simulink model "Final_Reciprocating_Simscape_19_08_24"  (R2023b)
settings: Solver=FixedStepAuto  StartTime=0.0  StopTime=T(end)  FixedStep=10^-4  RelTol=1e-3
values from neighbouring files (symbols this model uses):
  Kp1 = 10    [FFFB_PosForce_ME.m]    (also in FFFB_PosForce_ME1.m = 5000; FFFB_PosForce_ME2.m = 5000; FFFB_Posarbitary_actual_Mass.m = 5000; FFFB_arbitary_actual_Mass.m = 5000)
  Kp2 = 10000    [FFFB_PosForce_ME1.m]    (also in FFFB_PosForce_ME2.m; FFFB_Posarbitary_actual_Mass.m; FFFB_arbitary_actual_Mass.m; Kin_Trajectory_23_09_24.m)
  N = [-y1+y3;-x3+x1]    [Contact.m]
  X = 0.65    [Contact.m]    (also in FFFB_PosForce_ME.m = [X0',X1',X2']; FFFB_PosForce_ME1.m = [X2']; FFFB_PosForce_ME2.m = [X110,X2']; FFFB_Posarbitary_actual_Mass.m = [X110])
  Y = [Y0',Y1',Y2']    [FFFB_PosForce_ME.m]    (also in FFFB_PosForce_ME1.m = [Y2']; FFFB_PosForce_ME2.m = [Y110,Y2']; FFFB_Posarbitary_actual_Mass.m = [Y110]; FFFB_arbitary_actual_Mass.m = [Y2'])
undefined symbols (not defined in the file or in its folder): Z
libraries: sm_lib x24, nesl_utility x9, robotcorelib x1
settings Model: Creator=91996  LastModifiedBy=Dell
settings ExplorerConfigSet: InternalSimMechanicsExplorerSettings="<ExplorerConfiguration><canonicalview>default</canonicalview><AnimationSetting><BasePlaybackSpeed>1.0</BasePlaybackSpeed><PlaybackSpeedFactor>256.0</PlaybackSpeedFactor></AnimationSetting><TilePanel><TileInfo><Tiles Columns=\"1\" Count=\"1\" Rows=\"1\"><Column Weight=\"1\"/><Row Weight=\"1\"/><Tile Height=\"1\" Width=\"1\" X=\"0\" Y=\"0\"/></Tiles></TileInfo><SceneInfo><SceneViewer><BGColor><R>0.941176474094390869</R><G>0.941176474094390869</G><B>0.941176474094390869</B></BGColor><Camera><DoPerspective>off</DoPerspective><Position><X>0.490000009536743164</X><Y>-0.75</Y><Z>0.0764452517032630507</Z></Position><Center><X>0.490000009536743164</X><Y>0.25</Y><Z>0.0764452517032630507</Z></Center><Up><X>0</X><Y>-0</Y><Z>1</Z></Up><ViewLimDist>1</ViewLimDist><YLim>0.35683862030506136</YLim><XLim>0.73638515281135386</XLim></Camera></SceneViewer></SceneInfo></TilePanel><MechEditorPanel><Cameras/><GfxPanelCameraMap/><VideoCreator><PlaybackSpeedRatio>1.0</PlaybackSpeedRatio><FrameRate>30</FrameRate><VideoFormat>Motion JPEG AVI</VideoFormat><FrameSize>auto</FrameSize></VideoCreator></MechEditorPanel></ExplorerConfiguration>"

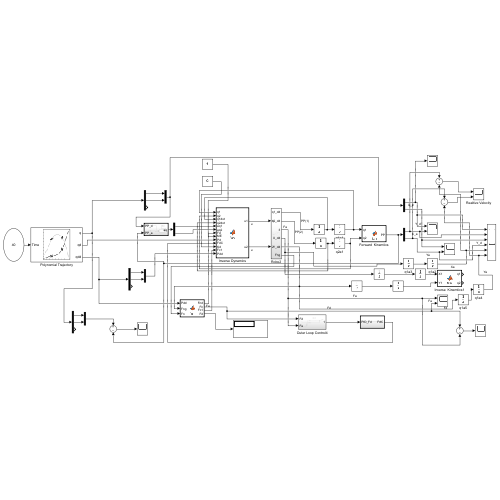
[thumbnail: Simulink's stored preview of the top-level diagram]
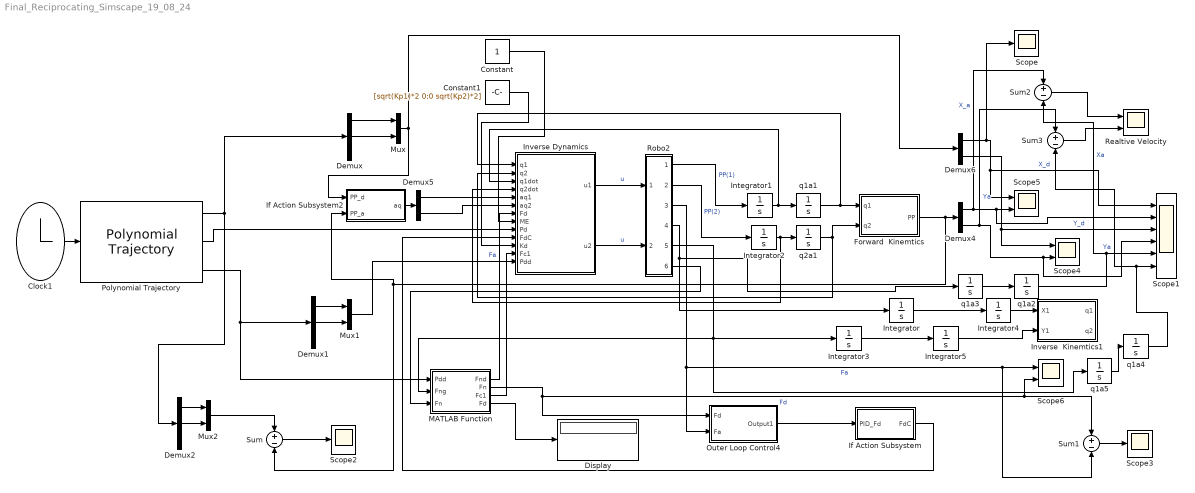
== system Final_Reciprocating_Simscape_19_08_24 ==
  Clock1 : Clock
  Constant : Constant
  Constant1 : Constant  Value=[sqrt(Kp1)*2 0;0 sqrt(Kp2)*2]
  Demux : Demux  Outputs=3
  Demux1 : Demux  Outputs=3
  Demux2 : Demux  Outputs=3
  Demux4 : Demux  Outputs=2
  Demux5 : Demux  Outputs=2
  Demux6 : Demux  Outputs=2
  Display : Display
  Forward  Kinemtics : MATLAB Function  TreatAsAtomicUnit=on
  If Action Subsystem : Subsystem  TreatAsAtomicUnit=on
  If Action Subsystem2 : Subsystem  TreatAsAtomicUnit=on
  Integrator{,1..5} (6 alike) : Integrator
  Inverse  Kinemtics1 : MATLAB Function  TreatAsAtomicUnit=on
  Inverse Dynamics : MATLAB Function  TreatAsAtomicUnit=on
  MATLAB Function : MATLAB Function  TreatAsAtomicUnit=on
  Mux : Mux  Inputs=2
  Mux1 : Mux  Inputs=2
  Mux2 : Mux  Inputs=2
  Outer Loop Control4 : Subsystem
  Polynomial Trajectory : robotcorelib/Polynomial Trajectory  WaypointSource=Internal  Waypoints=P  TimePoints=T  TimeInterval=[ 1, 4 ]  Method=Quintic Polynomial  ParameterSource=Internal  VelocityBoundaryCondition=Pd  AccelerationBoundaryCondition=Pdd  SimulateUsing=Interpreted execution
  Realtive Velocity : Scope  NumInputPorts=2
  Robo2 : Subsystem
  Scope : Scope
  Scope1 : Scope  NumInputPorts=6
  Scope2 : Scope
  Scope3 : Scope
  Scope4 : Scope  NumInputPorts=2
  Scope5 : Scope  NumInputPorts=2
  Scope6 : Scope  NumInputPorts=2
  Sum{,1..3} (4 alike) : Sum  Inputs=+-
  q1a1 : Integrator  InitialCondition=0.3778
  q1a2 : Integrator  InitialCondition=0.65
  q1a3 : Integrator
  q1a4 : Integrator  InitialCondition=0.2
  q1a5 : Integrator
  q2a1 : Integrator  InitialCondition=-1.5690
  wires:
  Inverse Dynamics/1(u1) -> Robo2/1(Input)  "u"
  Demux5/2 -> Inverse Dynamics/6(aq2)
  Demux6/2 -> Scope4/1, Scope1/3  "Y_d"
  Mux/1 -> If Action Subsystem2/1(PP_d), Demux6/1
  Integrator4/1 -> Inverse  Kinemtics1/1(X1)
  Robo2/5(Y_dd) -> q1a5/1, Integrator3/1, MATLAB Function/2(Fng)
  Demux/1 -> Mux/1
  Integrator/1 -> Integrator4/1
  Integrator3/1 -> Integrator5/1
  Integrator5/1 -> Inverse  Kinemtics1/2(Y1)
  Demux5/1 -> Inverse Dynamics/5(aq1)
  Polynomial Trajectory/3 -> MATLAB Function/1(Pdd), Demux1/1
  Demux4/1 -> Sum2/1, Scope1/2, Scope5/2  "X_a"
  If Action Subsystem2/1(aq) -> Demux5/1
  Clock1/1 -> Polynomial Trajectory/1
  q2a1/1 -> Forward  Kinemtics/2(q2), Inverse Dynamics/2(q2)
  Outer Loop Control4/1(Output1) -> If Action Subsystem/1(PID_Fd)
  Robo2/4(X_dd) -> q1a3/1, Integrator/1
  Integrator2/1 -> q2a1/1, Inverse Dynamics/4(q2dot)
  Demux6/1 -> Scope/1, Scope5/1, Scope1/1  "X_d"
  Inverse Dynamics/2(u2) -> Robo2/2(Input1)  "u"
  Integrator1/1 -> q1a1/1, Inverse Dynamics/3(q1dot)
  Robo2/2(q2_dd) -> Integrator2/1  "PP(2)"
  q1a1/1 -> Forward  Kinemtics/1(q1), Inverse Dynamics/1(q1)
  Robo2/1(q1_dd) -> Integrator1/1  "PP(1)"
  Demux/2 -> Mux/2
  Demux4/2 -> Scope1/4, Scope4/2, Sum3/1  "Ya"
  Constant/1 -> Inverse Dynamics/8(ME)
  Mux2/1 -> Sum/1
  Forward  Kinemtics/1(PP) -> Sum/2, If Action Subsystem2/2(PP_a), Demux4/1
  Sum/1 -> Scope2/1
  Demux2/2 -> Mux2/2
  Polynomial Trajectory/1 -> Demux/1, Demux2/1
  Demux2/1 -> Mux2/1
  MATLAB Function/2(Fn) -> Outer Loop Control4/1(Fd), Scope6/2, Sum1/1  "Fd"
  Sum1/1 -> Scope3/1
  Robo2/3(Output2) -> Outer Loop Control4/2(Fa), Scope6/1, Sum1/2  "Fa"
  Polynomial Trajectory/2 -> Inverse Dynamics/9(Pd)
  If Action Subsystem/1(FdC) -> Inverse Dynamics/10(FdC)
  Constant1/1 -> Inverse Dynamics/11(Kd)
  MATLAB Function/1(Fnd) -> Inverse Dynamics/7(Fd)  "Fa"
  MATLAB Function/3(Fc1) -> Inverse Dynamics/12(Fc1)
  Demux1/1 -> Mux1/1
  Demux1/2 -> Mux1/2
  Mux1/1 -> Inverse Dynamics/13(Pdd)
  Robo2/6(Fng) -> MATLAB Function/3("Fn ")
  MATLAB Function/4(Fd) -> Display/1
  q1a3/1 -> q1a2/1
  q1a2/1 -> Sum2/2, Scope1/5  "Xa"
  q1a5/1 -> q1a4/1
  q1a4/1 -> Sum3/2, Scope1/6  "Ya"
  Sum2/1 -> Realtive Velocity/1
  Sum3/1 -> Realtive Velocity/2

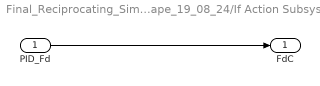
== system Final_Reciprocating_Simscape_19_08_24/If Action Subsystem ==
  PID_Fd : Inport
  FdC : Outport
  wires:
  PID_Fd/1 -> FdC/1

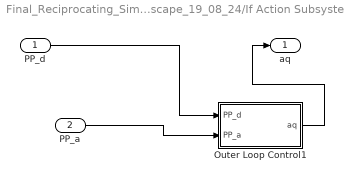
== system Final_Reciprocating_Simscape_19_08_24/If Action Subsystem2 ==
  PP_d : Inport
  PP_a : Inport  Port=2
  Outer Loop Control1 : Subsystem
  aq : Outport
  wires:
  PP_d/1 -> Outer Loop Control1/1(PP_d)
  Outer Loop Control1/1(aq) -> aq/1
  PP_a/1 -> Outer Loop Control1/2(PP_a)

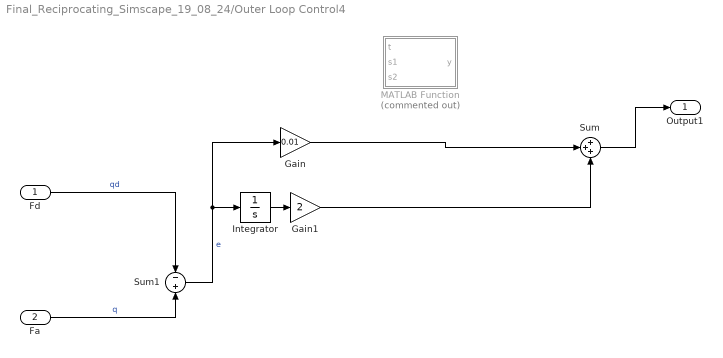
== system Final_Reciprocating_Simscape_19_08_24/Outer Loop Control4 ==
  Fd : Inport
  Fa : Inport  Port=2
  Gain : Gain  Gain=0.01
  Gain1 : Gain  Gain=2
  Integrator : Integrator
  MATLAB Function : MATLAB Function  Commented=on  TreatAsAtomicUnit=on
  Sum : Sum  Inputs=+++
  Sum1 : Sum  Inputs=-+
  Output1 : Outport
  wires:
  Sum1/1 -> Gain/1, Integrator/1  "e"
  Fd/1 -> Sum1/1  "qd"
  Fa/1 -> Sum1/2  "q"
  Integrator/1 -> Gain1/1
  Gain/1 -> Sum/2
  Gain1/1 -> Sum/3
  Sum/1 -> Output1/1

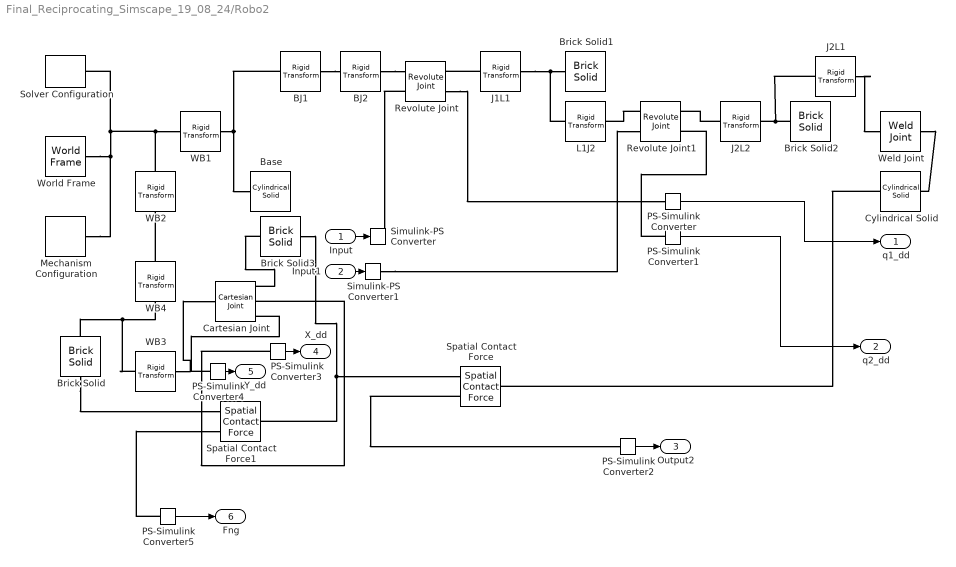
== system Final_Reciprocating_Simscape_19_08_24/Robo2 ==
  Input : Inport
  Input1 : Inport  Port=2
  BJ1 : sm_lib/Frames and Transforms/Rigid Transform  TranslationMethod=StandardAxis  TranslationStandardOffset=0.25  TranslationStandardOffsetUnits=m  TranslationStandardAxis=+Z  TranslationCartesianOffset=[0 0 0]  TranslationCartesianOffsetUnits=m  TranslationROffset=0  TranslationROffsetUnits=m  TranslationZOffset=0  TranslationZOffsetUnits=m  TranslationThetaOffset=0  TranslationThetaOffsetUnits=deg  RotationMethod=StandardAxis  RotationAngleUnits=deg  RotationStandardAxis=+X  RotationAngle=90  RotationArbitraryAxis=[0 0 1]  FollAlignAxisA=+X  BaseAlignAxisA=+Y  FollAlignAxisB=+Y  BaseAlignAxisB=+Z  RotationSequenceAxes=FollowerAxes  RotationSequence=XYX  RotationSequenceAngles=[0 0 0]  RotationSequenceAnglesUnits=deg  RotationMatrix=[1 0 0; 0 1 0; 0 0 1]  Quaternion=[1 0 0 0]
  BJ2 : sm_lib/Frames and Transforms/Rigid Transform  TranslationMethod=None  TranslationStandardOffset=0  TranslationStandardOffsetUnits=m  TranslationStandardAxis=+Z  TranslationCartesianOffset=[0 0 0]  TranslationCartesianOffsetUnits=m  TranslationROffset=0  TranslationROffsetUnits=m  TranslationZOffset=0  TranslationZOffsetUnits=m  TranslationThetaOffset=0  TranslationThetaOffsetUnits=deg  RotationMethod=StandardAxis  RotationAngleUnits=rad  RotationStandardAxis=+Z  RotationAngle=0.3778  RotationArbitraryAxis=[0 0 1]  FollAlignAxisA=+X  BaseAlignAxisA=+Y  FollAlignAxisB=+Y  BaseAlignAxisB=+Z  RotationSequenceAxes=FollowerAxes  RotationSequence=XYX  RotationSequenceAngles=[0 0 0]  RotationSequenceAnglesUnits=deg  RotationMatrix=[1 0 0; 0 1 0; 0 0 1]  Quaternion=[1 0 0 0]
  Base : sm_lib/Body Elements/Cylindrical Solid  GraphicAmbientColor=[0.15 0.15 0.15 1.0]  BasedOnType=Density  CenterOfMass=[0 0 0]  CenterOfMassUnits=m  GraphicDiffuseColor=[0.5 0.5 0.5]  CylinderLength=0.5  CylinderLengthUnits=m  CylinderRadius=0.02  CylinderRadiusUnits=m  Density=10000  DensityUnits=kg/m^3  DoExposeReferenceFrame=on  GraphicEmissiveColor=[0.0 0.0 0.0 1.0]  ExportEntireGeometry=off  SerializedFrames=<Frames/>  MarkerShape=Sphere  MarkerSize=10  GraphicType=FromGeometry  InertiaType=CalculateFromGeometry  Mass=1  MassUnits=kg  MomentsOfInertia=[1 1 1]  MomentsOfInertiaUnits=kg*m^2  GraphicOpacity=1.0  ProductsOfInertia=[0 0 0]  ProductsOfInertiaUnits=kg*m^2  GraphicShininess=75  GraphicSpecularColor=[0.5 0.5 0.5 1.0]  GraphicVisPropType=SimpleVisualProperties
  Brick Solid : sm_lib/Body Elements/Brick Solid  GraphicAmbientColor=[0.15 0.15 0.15 1.0]  BasedOnType=Density  BrickDimensions=[1 0.02 0.02]  BrickDimensionsUnits=m  CenterOfMass=[0 0 0]  CenterOfMassUnits=m  GraphicDiffuseColor=[0.5 0.5 0.5]  Density=10000  DensityUnits=kg/m^3  DoExposeReferenceFrame=on  GraphicEmissiveColor=[0.0 0.0 0.0 1.0]  ExportEntireGeometry=on  SerializedFrames=<Frames/>  MarkerShape=Sphere  MarkerSize=10  GraphicType=FromGeometry  InertiaType=CalculateFromGeometry  Mass=1  MassUnits=kg  MomentsOfInertia=[1 1 1]  MomentsOfInertiaUnits=kg*m^2  GraphicOpacity=1.0  ProductsOfInertia=[0 0 0]  ProductsOfInertiaUnits=kg*m^2  GraphicShininess=75  GraphicSpecularColor=[0.5 0.5 0.5 1.0]  GraphicVisPropType=SimpleVisualProperties
  Brick Solid1 : sm_lib/Body Elements/Brick Solid  GraphicAmbientColor=[0.15 0.15 0.15 1.0]  BasedOnType=Density  BrickDimensions=[0.5 0.02 0.02]  BrickDimensionsUnits=m  CenterOfMass=[0 0 0]  CenterOfMassUnits=m  GraphicDiffuseColor=[0.2 0.2 1.0]  Density=7800  DensityUnits=kg/m^3  DoExposeReferenceFrame=on  GraphicEmissiveColor=[0.0 0.0 0.0 1.0]  ExportEntireGeometry=off  SerializedFrames=<Frames/>  MarkerShape=Sphere  MarkerSize=10  GraphicType=FromGeometry  InertiaType=CalculateFromGeometry  Mass=1  MassUnits=kg  MomentsOfInertia=[1 1 1]  MomentsOfInertiaUnits=kg*m^2  GraphicOpacity=1.0  ProductsOfInertia=[0 0 0]  ProductsOfInertiaUnits=kg*m^2  GraphicShininess=75  GraphicSpecularColor=[0.5 0.5 0.5 1.0]  GraphicVisPropType=SimpleVisualProperties
  Brick Solid2 : sm_lib/Body Elements/Brick Solid  GraphicAmbientColor=[0.15 0.15 0.15 1.0]  BasedOnType=Density  BrickDimensions=[0.5 0.02 0.02]  BrickDimensionsUnits=m  CenterOfMass=[0 0 0]  CenterOfMassUnits=m  GraphicDiffuseColor=[0.0 0.8 0.2]  Density=7800  DensityUnits=kg/m^3  DoExposeReferenceFrame=on  GraphicEmissiveColor=[0.0 0.0 0.0 1.0]  ExportEntireGeometry=off  SerializedFrames=<Frames/>  MarkerShape=Sphere  MarkerSize=10  GraphicType=FromGeometry  InertiaType=CalculateFromGeometry  Mass=1  MassUnits=kg  MomentsOfInertia=[1 1 1]  MomentsOfInertiaUnits=kg*m^2  GraphicOpacity=1.0  ProductsOfInertia=[0 0 0]  ProductsOfInertiaUnits=kg*m^2  GraphicShininess=75  GraphicSpecularColor=[0.5 0.5 0.5 1.0]  GraphicVisPropType=SimpleVisualProperties
  Brick Solid3 : sm_lib/Body Elements/Brick Solid  GraphicAmbientColor=[0.15 0.15 0.15 1.0]  BasedOnType=Density  BrickDimensions=[0.22 0.02 0.2]  BrickDimensionsUnits=m  CenterOfMass=[0 0 0]  CenterOfMassUnits=m  GraphicDiffuseColor=[1.0 0.2 0.2]  Density=2000  DensityUnits=kg/m^3  DoExposeReferenceFrame=on  GraphicEmissiveColor=[0.0 0.0 0.0 1.0]  ExportEntireGeometry=on  SerializedFrames=<Frames/>  MarkerShape=Sphere  MarkerSize=10  GraphicType=FromGeometry  InertiaType=CalculateFromGeometry  Mass=1  MassUnits=kg  MomentsOfInertia=[1 1 1]  MomentsOfInertiaUnits=kg*m^2  GraphicOpacity=1.0  ProductsOfInertia=[0 0 0]  ProductsOfInertiaUnits=kg*m^2  GraphicShininess=75  GraphicSpecularColor=[0.5 0.5 0.5 1.0]  GraphicVisPropType=SimpleVisualProperties
  Cartesian Joint : sm_lib/Joints/Cartesian Joint  JointMode=Normal  SenseConstraintForce=off  SenseConstraintForceX=off  SenseConstraintForceY=off  SenseConstraintForceZ=off  SenseConstraintTorque=off  SenseConstraintTorqueX=off  SenseConstraintTorqueY=off  SenseConstraintTorqueZ=off  SenseTotalForce=off  SenseTotalForceX=off  SenseTotalForceY=off  SenseTotalForceZ=off  SenseTotalTorque=off  SenseTotalTorqueX=off  SenseTotalTorqueY=off  SenseTotalTorqueZ=off  CompositeWrenchDir=FollowerOnBase  CompositeWrenchFrame=BaseFrame  PxEquilibriumPosition=0  PxEquilibriumPositionUnits=m  PxSpringStiffness=0  PxSpringStiffnessUnits=N/m  PxDampingCoefficient=0  PxDampingCoefficientUnits=N/(m/s)  PxTorqueActuationMode=NoTorque  PxMotionActuationMode=ComputedMotion  PxSensePosition=off  PxSenseVelocity=off  PxSenseAcceleration=on  PxSenseTorqueForce=off  PxSenseLowerLimitTorqueForce=off  PxSenseUpperLimitTorqueForce=off  PxLowerLimitSpecify=off  PxLowerLimitBound=-1  PxLowerLimitBoundUnits=m  PxLowerLimitStiffness=1e6  PxLowerLimitStiffnessUnits=N/m  PxLowerLimitDamping=1e3  PxLowerLimitDampingUnits=N/(m/s)  PxLowerLimitTransitionRegionWidth=1e-4  PxLowerLimitTransitionRegionWidthUnits=m  PxUpperLimitSpecify=off  PxUpperLimitBound=1  PxUpperLimitBoundUnits=m  PxUpperLimitStiffness=1e6  PxUpperLimitStiffnessUnits=N/m  PxUpperLimitDamping=1e3  PxUpperLimitDampingUnits=N/(m/s)  PxUpperLimitTransitionRegionWidth=1e-4  PxUpperLimitTransitionRegionWidthUnits=m  PxPositionTargetSpecify=off  PxPositionTargetPriority=High  PxPositionTargetValue=0  PxPositionTargetValueUnits=m  PxVelocityTargetSpecify=off  PxVelocityTargetPriority=High  PxVelocityTargetValue=0  PxVelocityTargetValueUnits=m/s  PyEquilibriumPosition=0  PyEquilibriumPositionUnits=m  PySpringStiffness=0  PySpringStiffnessUnits=N/m  PyDampingCoefficient=0  PyDampingCoefficientUnits=N/(m/s)  PyTorqueActuationMode=NoTorque  PyMotionActuationMode=ComputedMotion  PySensePosition=off  PySenseVelocity=off  PySenseAcceleration=off  PySenseTorqueForce=off  PySenseLowerLimitTorqueForce=off  PySenseUpperLimitTorqueForce=off  PyLowerLimitSpecify=off  PyLowerLimitBound=-1  PyLowerLimitBoundUnits=m  PyLowerLimitStiffness=1e6  PyLowerLimitStiffnessUnits=N/m  PyLowerLimitDamping=1e3  PyLowerLimitDampingUnits=N/(m/s)  PyLowerLimitTransitionRegionWidth=1e-4  PyLowerLimitTransitionRegionWidthUnits=m  PyUpperLimitSpecify=off  PyUpperLimitBound=1  PyUpperLimitBoundUnits=m  PyUpperLimitStiffness=1e6  PyUpperLimitStiffnessUnits=N/m  PyUpperLimitDamping=1e3  PyUpperLimitDampingUnits=N/(m/s)  PyUpperLimitTransitionRegionWidth=1e-4  PyUpperLimitTransitionRegionWidthUnits=m  PyPositionTargetSpecify=off  PyPositionTargetPriority=High  PyPositionTargetValue=0  PyPositionTargetValueUnits=m  PyVelocityTargetSpecify=off  PyVelocityTargetPriority=High  PyVelocityTargetValue=0  PyVelocityTargetValueUnits=m/s  PzEquilibriumPosition=0  PzEquilibriumPositionUnits=m  PzSpringStiffness=0  PzSpringStiffnessUnits=N/m  PzDampingCoefficient=0  PzDampingCoefficientUnits=N/(m/s)  PzTorqueActuationMode=NoTorque  PzMotionActuationMode=ComputedMotion  PzSensePosition=off  PzSenseVelocity=off  PzSenseAcceleration=on  PzSenseTorqueForce=off  PzSenseLowerLimitTorqueForce=off  PzSenseUpperLimitTorqueForce=off  PzLowerLimitSpecify=off  PzLowerLimitBound=-1  PzLowerLimitBoundUnits=m  PzLowerLimitStiffness=1e6  PzLowerLimitStiffnessUnits=N/m  PzLowerLimitDamping=1e3  PzLowerLimitDampingUnits=N/(m/s)  PzLowerLimitTransitionRegionWidth=1e-4  PzLowerLimitTransitionRegionWidthUnits=m  PzUpperLimitSpecify=off  PzUpperLimitBound=1  PzUpperLimitBoundUnits=m  PzUpperLimitStiffness=1e6  PzUpperLimitStiffnessUnits=N/m  PzUpperLimitDamping=1e3  PzUpperLimitDampingUnits=N/(m/s)  PzUpperLimitTransitionRegionWidth=1e-4  PzUpperLimitTransitionRegionWidthUnits=m  PzPositionTargetSpecify=off  PzPositionTargetPriority=High  PzPositionTargetValue=0  PzPositionTargetValueUnits=m  PzVelocityTargetSpecify=off  PzVelocityTargetPriority=High  PzVelocityTargetValue=0  PzVelocityTargetValueUnits=m/s
  Cylindrical Solid : sm_lib/Body Elements/Cylindrical Solid  GraphicAmbientColor=[0.15 0.15 0.15 1.0]  BasedOnType=Density  CenterOfMass=[0 0 0]  CenterOfMassUnits=m  GraphicDiffuseColor=[0.5 0.5 0.5]  CylinderLength=0.02  CylinderLengthUnits=m  CylinderRadius=0.01  CylinderRadiusUnits=m  Density=7800  DensityUnits=kg/m^3  DoExposeReferenceFrame=on  GraphicEmissiveColor=[0.0 0.0 0.0 1.0]  ExportEntireGeometry=on  SerializedFrames=<Frames/>  MarkerShape=Sphere  MarkerSize=10  GraphicType=FromGeometry  InertiaType=CalculateFromGeometry  Mass=1  MassUnits=kg  MomentsOfInertia=[1 1 1]  MomentsOfInertiaUnits=kg*m^2  GraphicOpacity=1.0  ProductsOfInertia=[0 0 0]  ProductsOfInertiaUnits=kg*m^2  GraphicShininess=75  GraphicSpecularColor=[0.5 0.5 0.5 1.0]  GraphicVisPropType=SimpleVisualProperties
  J1L1 : sm_lib/Frames and Transforms/Rigid Transform  TranslationMethod=StandardAxis  TranslationStandardOffset=0.25  TranslationStandardOffsetUnits=m  TranslationStandardAxis=+X  TranslationCartesianOffset=[0 0 0]  TranslationCartesianOffsetUnits=m  TranslationROffset=0  TranslationROffsetUnits=m  TranslationZOffset=0  TranslationZOffsetUnits=m  TranslationThetaOffset=0  TranslationThetaOffsetUnits=deg  RotationMethod=None  RotationAngleUnits=deg  RotationStandardAxis=+Z  RotationAngle=0.0  RotationArbitraryAxis=[0 0 1]  FollAlignAxisA=+X  BaseAlignAxisA=+Y  FollAlignAxisB=+Y  BaseAlignAxisB=+Z  RotationSequenceAxes=FollowerAxes  RotationSequence=XYX  RotationSequenceAngles=[0 0 0]  RotationSequenceAnglesUnits=deg  RotationMatrix=[1 0 0; 0 1 0; 0 0 1]  Quaternion=[1 0 0 0]
  J2L1 : sm_lib/Frames and Transforms/Rigid Transform  TranslationMethod=StandardAxis  TranslationStandardOffset=(0.5)/2  TranslationStandardOffsetUnits=m  TranslationStandardAxis=+X  TranslationCartesianOffset=[0 0 0]  TranslationCartesianOffsetUnits=m  TranslationROffset=0  TranslationROffsetUnits=m  TranslationZOffset=0  TranslationZOffsetUnits=m  TranslationThetaOffset=0  TranslationThetaOffsetUnits=deg  RotationMethod=None  RotationAngleUnits=deg  RotationStandardAxis=+Z  RotationAngle=0.0  RotationArbitraryAxis=[0 0 1]  FollAlignAxisA=+X  BaseAlignAxisA=+Y  FollAlignAxisB=+Y  BaseAlignAxisB=+Z  RotationSequenceAxes=FollowerAxes  RotationSequence=XYX  RotationSequenceAngles=[0 0 0]  RotationSequenceAnglesUnits=deg  RotationMatrix=[1 0 0; 0 1 0; 0 0 1]  Quaternion=[1 0 0 0]
  J2L2 : sm_lib/Frames and Transforms/Rigid Transform  TranslationMethod=StandardAxis  TranslationStandardOffset=(0.5)/2  TranslationStandardOffsetUnits=m  TranslationStandardAxis=+X  TranslationCartesianOffset=[0 0 0]  TranslationCartesianOffsetUnits=m  TranslationROffset=0  TranslationROffsetUnits=m  TranslationZOffset=0  TranslationZOffsetUnits=m  TranslationThetaOffset=0  TranslationThetaOffsetUnits=deg  RotationMethod=None  RotationAngleUnits=deg  RotationStandardAxis=+Z  RotationAngle=0.0  RotationArbitraryAxis=[0 0 1]  FollAlignAxisA=+X  BaseAlignAxisA=+Y  FollAlignAxisB=+Y  BaseAlignAxisB=+Z  RotationSequenceAxes=FollowerAxes  RotationSequence=XYX  RotationSequenceAngles=[0 0 0]  RotationSequenceAnglesUnits=deg  RotationMatrix=[1 0 0; 0 1 0; 0 0 1]  Quaternion=[1 0 0 0]
  L1J2 : sm_lib/Frames and Transforms/Rigid Transform  TranslationMethod=StandardAxis  TranslationStandardOffset=0.25  TranslationStandardOffsetUnits=m  TranslationStandardAxis=+X  TranslationCartesianOffset=[0 0 0]  TranslationCartesianOffsetUnits=m  TranslationROffset=0  TranslationROffsetUnits=m  TranslationZOffset=0  TranslationZOffsetUnits=m  TranslationThetaOffset=0  TranslationThetaOffsetUnits=deg  RotationMethod=StandardAxis  RotationAngleUnits=rad  RotationStandardAxis=+Z  RotationAngle=-1.5690  RotationArbitraryAxis=[0 0 1]  FollAlignAxisA=+X  BaseAlignAxisA=+Y  FollAlignAxisB=+Y  BaseAlignAxisB=+Z  RotationSequenceAxes=FollowerAxes  RotationSequence=XYX  RotationSequenceAngles=[0 0 0]  RotationSequenceAnglesUnits=deg  RotationMatrix=[1 0 0; 0 1 0; 0 0 1]  Quaternion=[1 0 0 0]
  Mechanism Configuration : sm_lib/Utilities/Mechanism Configuration  UniformGravity=Constant  GravityVector=[0 0 -9.80665]  GravityVectorUnits=m/s^2  LinearizationDelta=0.001  JointModeTransitionNonlinearIterations=2
  PS-Simulink Converter{,1..5} (6 alike) : nesl_utility/PS-Simulink Converter  PhysicalDomain=network_engine_domain  SubClassName=ps_output  LeftPortType=input  RightPortType=output  PseudoPeriodic=off  Frequencies=[]  VectorFormat=inherit  Unit=inherit  AffineConversion=off
  Revolute Joint : sm_lib/Joints/Revolute Joint  JointMode=Normal  SenseConstraintForce=off  SenseConstraintForceX=off  SenseConstraintForceY=off  SenseConstraintForceZ=off  SenseConstraintTorque=off  SenseConstraintTorqueX=off  SenseConstraintTorqueY=off  SenseConstraintTorqueZ=off  SenseTotalForce=off  SenseTotalForceX=off  SenseTotalForceY=off  SenseTotalForceZ=off  SenseTotalTorque=off  SenseTotalTorqueX=off  SenseTotalTorqueY=off  SenseTotalTorqueZ=off  CompositeWrenchDir=FollowerOnBase  CompositeWrenchFrame=BaseFrame  EquilibriumPosition=0  EquilibriumPositionUnits=deg  SpringStiffness=0  SpringStiffnessUnits=N*m/deg  DampingCoefficient=0  DampingCoefficientUnits=N*m/(deg/s)  TorqueActuationMode=InputTorque  MotionActuationMode=ComputedMotion  SensePosition=off  SenseVelocity=off  SenseAcceleration=on  SenseTorqueForce=off  SenseLowerLimitTorqueForce=off  SenseUpperLimitTorqueForce=off  LowerLimitSpecify=off  LowerLimitBound=-90  LowerLimitBoundUnits=deg  LowerLimitStiffness=1e4  LowerLimitStiffnessUnits=N*m/deg  LowerLimitDamping=10  LowerLimitDampingUnits=N*m/(deg/s)  LowerLimitTransitionRegionWidth=0.1  LowerLimitTransitionRegionWidthUnits=deg  UpperLimitSpecify=off  UpperLimitBound=90  UpperLimitBoundUnits=deg  UpperLimitStiffness=1e4  UpperLimitStiffnessUnits=N*m/deg  UpperLimitDamping=10  UpperLimitDampingUnits=N*m/(deg/s)  UpperLimitTransitionRegionWidth=0.1  UpperLimitTransitionRegionWidthUnits=deg  PositionTargetSpecify=off  PositionTargetPriority=High  PositionTargetValue=0  PositionTargetValueUnits=deg  VelocityTargetSpecify=off  VelocityTargetPriority=High  VelocityTargetValue=0  VelocityTargetValueUnits=deg/s
  Revolute Joint1 : sm_lib/Joints/Revolute Joint  JointMode=Normal  SenseConstraintForce=off  SenseConstraintForceX=off  SenseConstraintForceY=off  SenseConstraintForceZ=off  SenseConstraintTorque=off  SenseConstraintTorqueX=off  SenseConstraintTorqueY=off  SenseConstraintTorqueZ=off  SenseTotalForce=off  SenseTotalForceX=off  SenseTotalForceY=off  SenseTotalForceZ=off  SenseTotalTorque=off  SenseTotalTorqueX=off  SenseTotalTorqueY=off  SenseTotalTorqueZ=off  CompositeWrenchDir=FollowerOnBase  CompositeWrenchFrame=BaseFrame  EquilibriumPosition=0  EquilibriumPositionUnits=deg  SpringStiffness=0  SpringStiffnessUnits=N*m/deg  DampingCoefficient=0  DampingCoefficientUnits=N*m/(deg/s)  TorqueActuationMode=InputTorque  MotionActuationMode=ComputedMotion  SensePosition=off  SenseVelocity=off  SenseAcceleration=on  SenseTorqueForce=off  SenseLowerLimitTorqueForce=off  SenseUpperLimitTorqueForce=off  LowerLimitSpecify=off  LowerLimitBound=-90  LowerLimitBoundUnits=deg  LowerLimitStiffness=1e4  LowerLimitStiffnessUnits=N*m/deg  LowerLimitDamping=10  LowerLimitDampingUnits=N*m/(deg/s)  LowerLimitTransitionRegionWidth=0.1  LowerLimitTransitionRegionWidthUnits=deg  UpperLimitSpecify=off  UpperLimitBound=90  UpperLimitBoundUnits=deg  UpperLimitStiffness=1e4  UpperLimitStiffnessUnits=N*m/deg  UpperLimitDamping=10  UpperLimitDampingUnits=N*m/(deg/s)  UpperLimitTransitionRegionWidth=0.1  UpperLimitTransitionRegionWidthUnits=deg  PositionTargetSpecify=off  PositionTargetPriority=High  PositionTargetValue=0  PositionTargetValueUnits=deg  VelocityTargetSpecify=off  VelocityTargetPriority=High  VelocityTargetValue=0  VelocityTargetValueUnits=deg/s
  Simulink-PS Converter : nesl_utility/Simulink-PS Converter  PhysicalDomain=network_engine_domain  SubClassName=ps_input  LeftPortType=input  RightPortType=output  PseudoPeriodic=off  Frequencies=[]  NoiseDistribution=none  NoiseParameters=[]  Unit=N*m  AffineConversion=off  FilteringAndDerivatives=provide  SimscapeFilterOrder=1  InputFilterTimeConstant=0.001  UdotUserProvided=0
  Simulink-PS Converter1 : nesl_utility/Simulink-PS Converter  PhysicalDomain=network_engine_domain  SubClassName=ps_input  LeftPortType=input  RightPortType=output  PseudoPeriodic=off  Frequencies=[]  NoiseDistribution=none  NoiseParameters=[]  Unit=N*m  AffineConversion=off  FilteringAndDerivatives=provide  SimscapeFilterOrder=1  InputFilterTimeConstant=0.001  UdotUserProvided=0
  Solver Configuration : nesl_utility/Solver Configuration  PhysicalDomain=network_engine_domain  SubClassName=solver  LeftPortType=input  RightPortType=generic  Tones=[]  Harmonics=[]  SimulateNoise=off  Profile=off  UseLocalSampling=off  EnableSwitchedLinearOptims=on  FrequencyDomain=off  UseCCode=off  RelTol=0.001  AbsTol=1e-06  MinStep=1e-09  ToWorkspace=off  RevertToSquareIcSolve=off  NumHomotopyIterations=100  PhasorMode=off  PhasorModeNumHarmonics=1  ConsistencySolver=NEWTON_XTOL_AFTER_FTOL  IndexReductionMethod=DerivativeReplacement  DoDC=off  ResidualTolerance=1e-09  ConsistencyTolSource=GLOBAL  ConsistencyAbsTol=0.001  ConsistencyRelTol=0.001  ConsistencyTolFactor=0.001  UseLocalSolver=off  LocalSolverChoice=NE_BACKWARD_EULER_ADVANCER  ResolveIndetEquations=on  FunctionEvalNumThread=1  LocalSolverSampleTime=0.001  DoFixedCost=off  MaxNonlinIter=3  MaxModeIter=2  ComputeImpulses=off  ImpulseIterations=2  LinearAlgebra=Sparse  LinearAlgebraNumThread=0  EquationFormulation=NE_TIME_EF  DelaysMemoryBudget=1024  AutomaticFiltering=on  FilteringTimeConstant=0.001  PartitionStorageMethod=AS_NEEDED  PartitionMemoryBudget=1024  PartitionMethod=FAST  MultibodyUseLocalSolver=off  MultibodyLocalSolverChoice=ODE1  MultibodyLocalSolverSampleTime=0.001
  Spatial Contact Force : sm_lib/Forces and Torques/Spatial Contact Force  SenseContactBaseRotation=off  SenseContactBaseTranslation=off  CoefficientOfDynamicFriction=0.3  CoefficientOfStaticFriction=0.5  NormalDamping=1e6  NormalDampingUnits=N/(m/s)  SenseContactSignal=off  NormalStiffness=1e6  NormalStiffnessUnits=N/m  FrictionalCriticalVelocity=1e-3  FrictionalCriticalVelocityUnits=m/s  ZeroCrossDetectContactStartAndEnd=off  SenseContactFollowerRotation=off  SenseContactFollowerTranslation=off  FrictionType=SmoothStickSlip  SenseFrictionalForceMagnitude=off  SenseNormalForceMagnitude=on  NormalForceType=SmoothSpringDamper  SenseNormalVelocity=off  SensePenetrationDepth=off  SenseSeparationDistance=off  SenseTangentialVelocity=off  NormalTransitionRegionWidth=1e-4  NormalTransitionRegionWidthUnits=m
  Spatial Contact Force1 : sm_lib/Forces and Torques/Spatial Contact Force  SenseContactBaseRotation=off  SenseContactBaseTranslation=off  CoefficientOfDynamicFriction=0.05  CoefficientOfStaticFriction=0.1  NormalDamping=1e6  NormalDampingUnits=N/(m/s)  SenseContactSignal=off  NormalStiffness=1e6  NormalStiffnessUnits=N/m  FrictionalCriticalVelocity=1e-3  FrictionalCriticalVelocityUnits=m/s  ZeroCrossDetectContactStartAndEnd=off  SenseContactFollowerRotation=off  SenseContactFollowerTranslation=off  FrictionType=SmoothStickSlip  SenseFrictionalForceMagnitude=off  SenseNormalForceMagnitude=on  NormalForceType=SmoothSpringDamper  SenseNormalVelocity=off  SensePenetrationDepth=off  SenseSeparationDistance=off  SenseTangentialVelocity=off  NormalTransitionRegionWidth=1e-4  NormalTransitionRegionWidthUnits=m
  WB1 : sm_lib/Frames and Transforms/Rigid Transform  TranslationMethod=Cartesian  TranslationStandardOffset=0  TranslationStandardOffsetUnits=m  TranslationStandardAxis=+Z  TranslationCartesianOffset=[0 0.25 0]  TranslationCartesianOffsetUnits=m  TranslationROffset=0  TranslationROffsetUnits=m  TranslationZOffset=0  TranslationZOffsetUnits=m  TranslationThetaOffset=0  TranslationThetaOffsetUnits=deg  RotationMethod=None  RotationAngleUnits=deg  RotationStandardAxis=+X  RotationAngle=90  RotationArbitraryAxis=[0 0 1]  FollAlignAxisA=+X  BaseAlignAxisA=+Y  FollAlignAxisB=+Y  BaseAlignAxisB=+Z  RotationSequenceAxes=FollowerAxes  RotationSequence=XYX  RotationSequenceAngles=[0 0 0]  RotationSequenceAnglesUnits=deg  RotationMatrix=[1 0 0; 0 1 0; 0 0 1]  Quaternion=[1 0 0 0]
  WB2 : sm_lib/Frames and Transforms/Rigid Transform  TranslationMethod=Cartesian  TranslationStandardOffset=0  TranslationStandardOffsetUnits=m  TranslationStandardAxis=+Z  TranslationCartesianOffset="[-0.5   -0.25  0.25 ]"  TranslationCartesianOffsetUnits=m  TranslationROffset=0  TranslationROffsetUnits=m  TranslationZOffset=0  TranslationZOffsetUnits=m  TranslationThetaOffset=0  TranslationThetaOffsetUnits=deg  RotationMethod=None  RotationAngleUnits=deg  RotationStandardAxis=+X  RotationAngle=90  RotationArbitraryAxis=[0 0 1]  FollAlignAxisA=+X  BaseAlignAxisA=+Y  FollAlignAxisB=+Y  BaseAlignAxisB=+Z  RotationSequenceAxes=FollowerAxes  RotationSequence=XYX  RotationSequenceAngles=[0 0 0]  RotationSequenceAnglesUnits=deg  RotationMatrix=[1 0 0; 0 1 0; 0 0 1]  Quaternion=[1 0 0 0]
  WB3 : sm_lib/Frames and Transforms/Rigid Transform  TranslationMethod=Cartesian  TranslationStandardOffset=0  TranslationStandardOffsetUnits=m  TranslationStandardAxis=+Z  TranslationCartesianOffset="[-0.25  0  -0.1-0.01 ]"  TranslationCartesianOffsetUnits=m  TranslationROffset=0  TranslationROffsetUnits=m  TranslationZOffset=0  TranslationZOffsetUnits=m  TranslationThetaOffset=0  TranslationThetaOffsetUnits=deg  RotationMethod=None  RotationAngleUnits=deg  RotationStandardAxis=+X  RotationAngle=90  RotationArbitraryAxis=[0 0 1]  FollAlignAxisA=+X  BaseAlignAxisA=+Y  FollAlignAxisB=+Y  BaseAlignAxisB=+Z  RotationSequenceAxes=FollowerAxes  RotationSequence=XYX  RotationSequenceAngles=[0 0 0]  RotationSequenceAnglesUnits=deg  RotationMatrix=[1 0 0; 0 1 0; 0 0 1]  Quaternion=[1 0 0 0]
  WB4 : sm_lib/Frames and Transforms/Rigid Transform  TranslationMethod=Cartesian  TranslationStandardOffset=0  TranslationStandardOffsetUnits=m  TranslationStandardAxis=+Z  TranslationCartesianOffset=[0,0,0.01 ]  TranslationCartesianOffsetUnits=m  TranslationROffset=0  TranslationROffsetUnits=m  TranslationZOffset=0  TranslationZOffsetUnits=m  TranslationThetaOffset=0  TranslationThetaOffsetUnits=deg  RotationMethod=None  RotationAngleUnits=deg  RotationStandardAxis=+X  RotationAngle=90  RotationArbitraryAxis=[0 0 1]  FollAlignAxisA=+X  BaseAlignAxisA=+Y  FollAlignAxisB=+Y  BaseAlignAxisB=+Z  RotationSequenceAxes=FollowerAxes  RotationSequence=XYX  RotationSequenceAngles=[0 0 0]  RotationSequenceAnglesUnits=deg  RotationMatrix=[1 0 0; 0 1 0; 0 0 1]  Quaternion=[1 0 0 0]
  Weld Joint : sm_lib/Joints/Weld Joint  JointMode=Normal  SenseConstraintForce=off  SenseConstraintForceX=off  SenseConstraintForceY=off  SenseConstraintForceZ=off  SenseConstraintTorque=off  SenseConstraintTorqueX=off  SenseConstraintTorqueY=off  SenseConstraintTorqueZ=off  SenseTotalForce=off  SenseTotalForceX=off  SenseTotalForceY=off  SenseTotalForceZ=off  SenseTotalTorque=off  SenseTotalTorqueX=off  SenseTotalTorqueY=off  SenseTotalTorqueZ=off  CompositeWrenchDir=FollowerOnBase  CompositeWrenchFrame=BaseFrame
  World Frame : sm_lib/Frames and Transforms/World Frame
  q1_dd : Outport
  q2_dd : Outport  Port=2
  Output2 : Outport  Port=3
  X_dd : Outport  Port=4
  Y_dd : Outport  Port=5
  Fng : Outport  Port=6
  wires:
  Input/1 -> Simulink-PS Converter/1
  Input1/1 -> Simulink-PS Converter1/1
  PS-Simulink Converter/1 -> q1_dd/1
  PS-Simulink Converter1/1 -> q2_dd/1
  PS-Simulink Converter2/1 -> Output2/1
  PS-Simulink Converter3/1 -> X_dd/1
  PS-Simulink Converter4/1 -> Y_dd/1
  PS-Simulink Converter5/1 -> Fng/1
  connections:
  BJ1/LConn1 -- Base/RConn1 -- WB1/RConn1
  J1L1/RConn1 -- L1J2/LConn1 -- Brick Solid1/RConn1
  Revolute Joint1/LConn1 -- L1J2/RConn1
  Brick Solid2/RConn1 -- J2L1/LConn1 -- J2L2/RConn1
  J1L1/LConn1 -- Revolute Joint/RConn1
  J2L2/LConn1 -- Revolute Joint1/RConn1
  Revolute Joint/LConn2 -- Simulink-PS Converter/RConn1
  Simulink-PS Converter1/RConn1 -- Revolute Joint1/LConn2
  Revolute Joint/RConn2 -- PS-Simulink Converter/LConn1
  PS-Simulink Converter1/LConn1 -- Revolute Joint1/RConn2
  Solver Configuration/RConn1 -- WB2/RConn1 -- WB1/LConn1 -- Mechanism Configuration/RConn1 -- World Frame/RConn1
  WB4/RConn1 -- WB2/LConn1
  J2L1/RConn1 -- Weld Joint/LConn1
  Weld Joint/RConn1 -- Cylindrical Solid/RConn1
  BJ2/RConn1 -- Revolute Joint/LConn1
  WB4/LConn1 -- Brick Solid/RConn1 -- WB3/RConn1
  Spatial Contact Force/RConn2 -- PS-Simulink Converter2/LConn1
  BJ1/RConn1 -- BJ2/LConn1
  Brick Solid3/LConn1 -- Spatial Contact Force1/LConn1 -- Spatial Contact Force/RConn1
  Cylindrical Solid/LConn1 -- Spatial Contact Force/LConn1
  Brick Solid/LConn1 -- Spatial Contact Force1/RConn1
  WB3/LConn1 -- Cartesian Joint/LConn1
  Brick Solid3/RConn1 -- Cartesian Joint/RConn1
  PS-Simulink Converter3/LConn1 -- Cartesian Joint/RConn2
  PS-Simulink Converter4/LConn1 -- Cartesian Joint/RConn3
  PS-Simulink Converter5/LConn1 -- Spatial Contact Force1/RConn2

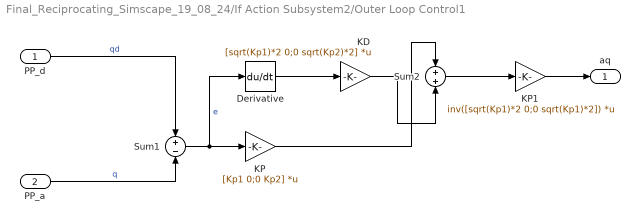
== system Final_Reciprocating_Simscape_19_08_24/If Action Subsystem2/Outer Loop Control1 ==
  PP_d : Inport
  PP_a : Inport  Port=2
  Derivative : Derivative
  KD : Gain  Gain=[sqrt(Kp1)*2 0;0 sqrt(Kp2)*2]  Multiplication=Matrix(K*u)
  KP : Gain  Gain=[Kp1 0;0 Kp2]  Multiplication=Matrix(K*u)
  KP1 : Gain  Gain=inv([sqrt(Kp1)*2 0;0 sqrt(Kp1)*2])  Multiplication=Matrix(K*u)
  Sum1 : Sum  Inputs=+-
  Sum2 : Sum
  aq : Outport
  wires:
  KD/1 -> Sum2/2
  KP/1 -> Sum2/1
  Sum1/1 -> Derivative/1, KP/1  "e"
  Derivative/1 -> KD/1
  PP_d/1 -> Sum1/1  "qd"
  PP_a/1 -> Sum1/2  "q"
  Sum2/1 -> KP1/1
  KP1/1 -> aq/1

== matlab function Final_Reciprocating_Simscape_19_08_24/Outer Loop Control4/MATLAB Function ==
  data: t input; y output; s1 input; s2 input
function y = fcn(t,s1,s2)
B=F0;

Kfp=0.01;
Kfi=-(Kfp)*log((s2/B))/(t+0.001);
y=real(s1*Kfi+s2*Kfi);

== matlab function Final_Reciprocating_Simscape_19_08_24/MATLAB Function ==
  data: Fnd output; Pdd input; Fn output; Fng input; Fc1 output; Fn input; Fd output
function [Fnd,Fn,Fc1,Fd]= fcn(Pdd,Fng,Fn)

mu=0.3;
mo=1.8;
Mo=[mo 0;0 mo];
g=-9.81;
Mu=mu;
Fd=Mo*[Pdd(1);Pdd(2)]+[Mu*(mo*g+Fn);0];
mus=0.5;
Fnd=Fd(1)/mus;
Fn=Fnd;
Fc1=[Fd(1);Fn];

== matlab function Final_Reciprocating_Simscape_19_08_24/Inverse  Kinemtics1 ==
  data: X1 input; q1 output; Y1 input; q2 output
function [q1,q2]= fcn(X1,Y1)
a1=0.5;
a2=0.5;
L01=0.5;
Z0=[1,2]';r=0.01;
for n=1:100
    q1=Z0(1);
    q2=Z0(2);
PP=R_EQ(L01,a1,a2,0,r,q1,q2)-[X1;Y1];
Jac = R_Jac1(a1,a2,q1,q2);

Z1=inv(Jac)*PP;
err=abs(Z1-Z0);
if err<=0.0001
    break
else Z0=Z1;
end
end

== matlab function Final_Reciprocating_Simscape_19_08_24/Inverse Dynamics ==
  data: q1 input; u1 output; q2 input; q1dot input; q2dot input; aq1 input; aq2 input; u2 output; Fd input; ME input; Pd input; FdC input; Kd input; Fc1 input; Pdd input
function [u1,u2] = fcn(q1,q2,q1dot,q2dot,aq1,aq2,Fd,ME,Pd,FdC,Kd,Fc1,Pdd)
% q2=q2-0.1;
g=-9.81;
a1=0.5;  
a2=0.5; 
L01=0.5;
m1=1.56*ME;
m2=1.5288*ME;
m3=0.0490088*ME;
C1=a1/2;
C2=(m2*0.5*a2+m3*a2)/(m2+m3);
Itot1=0.032552;
Itot2=0.0306397+2.45044e-06;
Jac = R_Jac1(a1,a2,q1,q2);
Jd=R_Jd1(a1,a2,q1,q2,q1dot,q2dot);
M=R_M(C1,C2,Itot1,Itot2,a1,m1,m2+m3,q2);
C = R_damp(C2,a1,m2+m3,q2,q1dot,q2dot);
G= R_Gra(C1,C2,a1,m1,m2+m3,g,q1,q2);
mus=0.5;
u=M*inv(Jac)*Pdd-M*inv(Jac)*Jd*[q1dot,q2dot]'+C+G+Jac'*Fc1+Kd*inv(Jac)*([aq1;aq2]);
u1=u(1);
u2=u(2);

== matlab function Final_Reciprocating_Simscape_19_08_24/Forward  Kinemtics ==
  data: q1 input; PP output; q2 input
function PP = fcn(q1,q2)
a1=0.5;
a2=0.5;
L01=0.5;
r=0.01;
PP=R_EQ(L01,a1,a2,0,r,q1,q2);
